simulink model "experiment1_h2_2"  (R2022b)
settings: Solver=VariableStepAuto  StartTime=0.0  StopTime=100.0  RelTol=1e-3
settings Model: Creator=lenovo  LastModifiedBy=acer
settings ModelReferenceCC: EnableRefExpFcnMdlSchedulingChecks=on

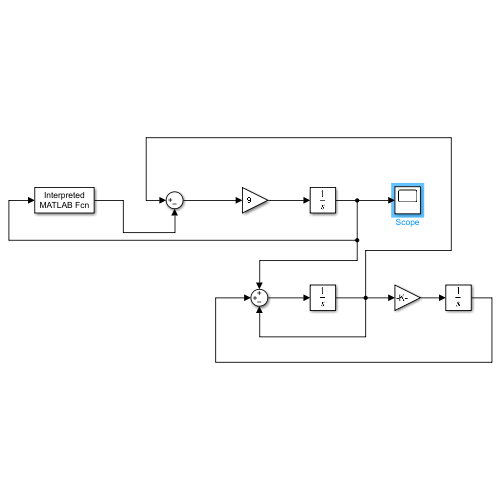
[thumbnail: Simulink's stored preview of the top-level diagram]
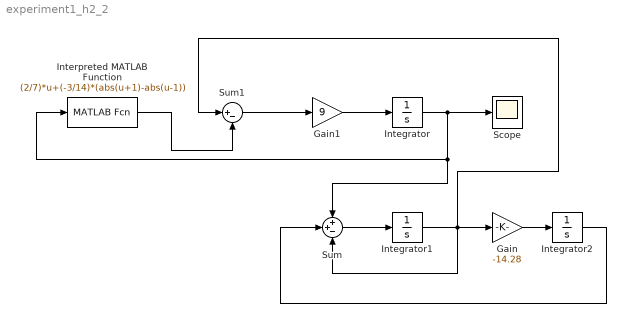
== system experiment1_h2_2 ==
  Gain : Gain  Gain=-14.28
  Gain1 : Gain  Gain=9
  Integrator : Integrator  InitialCondition=-0.2
  Integrator1 : Integrator  InitialCondition=0.3
  Integrator2 : Integrator  InitialCondition=0.7
  Interpreted MATLAB Function : MATLABFcn  MATLABFcn=(2/7)*u+(-3/14)*(abs(u+1)-abs(u-1))
  Scope : Scope
  Sum : Sum  Inputs=++-
  Sum1 : Sum  Inputs=|+-
  wires:
  Integrator/1 -> Sum/1, Interpreted MATLAB Function/1, Scope/1
  Integrator1/1 -> Sum/3, Sum1/1, Gain/1
  Gain/1 -> Integrator2/1
  Integrator2/1 -> Sum/2
  Sum/1 -> Integrator1/1
  Interpreted MATLAB Function/1 -> Sum1/2
  Sum1/1 -> Gain1/1
  Gain1/1 -> Integrator/1
